simulink model "giaihept"  (R2016a)
settings: Solver=VariableStepAuto  StartTime=0.0  StopTime=10.0  RelTol=1e-3
settings Model: Creator=cloud  LastModifiedBy=cloud

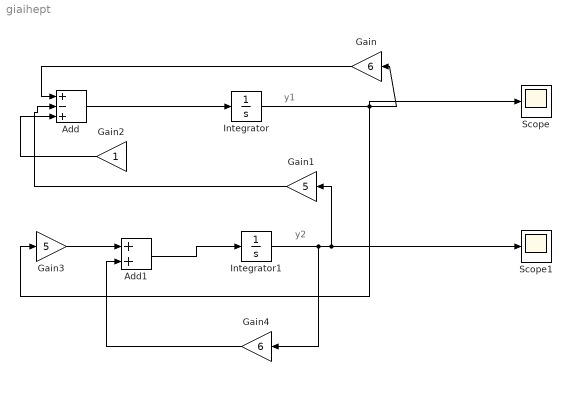
== system giaihept ==
  note: y2
  note: y1
  Add : Sum  Inputs=+-+
  Add1 : Sum
  Gain : Gain  Gain=6
  Gain1 : Gain  Gain=5
  Gain2 : Gain
  Gain3 : Gain  Gain=5
  Gain4 : Gain  Gain=6
  Integrator : Integrator
  Integrator1 : Integrator
  Scope : Scope
  Scope1 : Scope
  wires:
  Integrator/1 -> Scope/1, Gain3/1, Gain/1
  Gain/1 -> Add/1
  Integrator1/1 -> Scope1/1, Gain1/1, Gain4/1
  Gain1/1 -> Add/2
  Gain2/1 -> Add/3
  Add/1 -> Integrator/1
  Add1/1 -> Integrator1/1
  Gain3/1 -> Add1/1
  Gain4/1 -> Add1/2
